simulink model "Question3cd"  (R2023b)
settings: Solver=VariableStepAuto  StartTime=0.0  StopTime=60.0  RelTol=1e-3
settings Model: Creator=akank  LastModifiedBy=akank

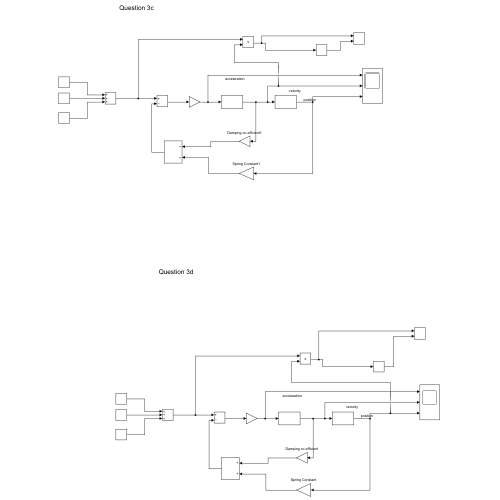
[thumbnail: Simulink's stored preview of the top-level diagram]
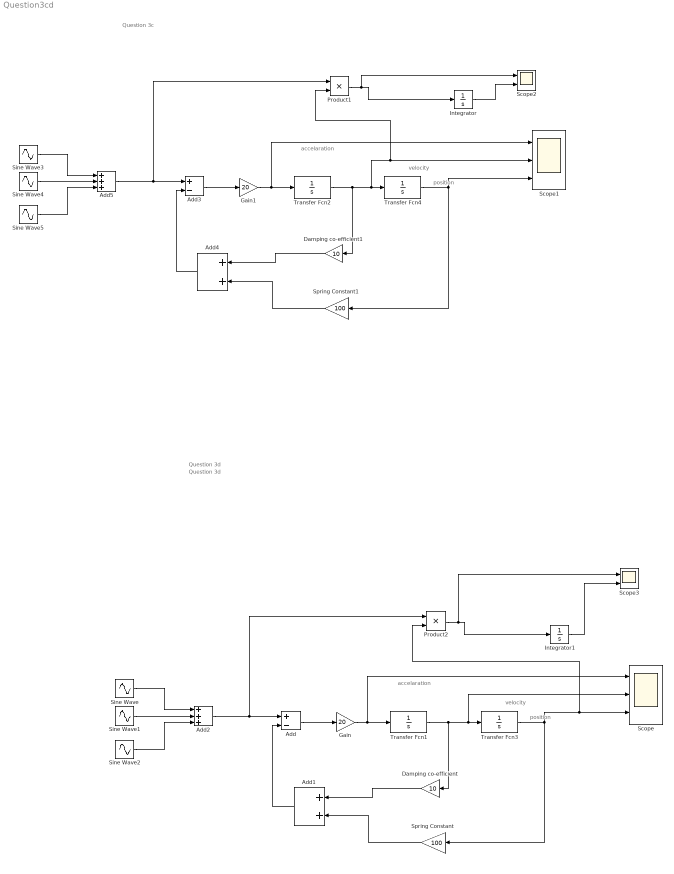
== system Question3cd ==
  note: Question 3c
  note: velocity
  note: accelaration
  note: position
  note: accelaration
  note: velocity
  note: position
  note: Question 3d
  note: Question 3d
  Add : Sum  Inputs=+-
  Add1 : Sum
  Add2 : Sum  Inputs=+++
  Add3 : Sum  Inputs=+-
  Add4 : Sum
  Add5 : Sum  Inputs=+++
  Damping co-efficient : Gain  Gain=10
  Damping co-efficient1 : Gain  Gain=10
  Gain : Gain  Gain=20
  Gain1 : Gain  Gain=20
  Integrator : Integrator  LimitOutput=on  LowerSaturationLimit=0
  Integrator1 : Integrator  LimitOutput=on  LowerSaturationLimit=0
  Product1 : Product
  Product2 : Product
  Scope : Scope  NumInputPorts=3
  Scope1 : Scope  NumInputPorts=3
  Scope2 : Scope  NumInputPorts=2
  Scope3 : Scope  NumInputPorts=2
  Sine Wave : Sin  Amplitude=20  SampleTime=0
  Sine Wave1 : Sin  Amplitude=10  Frequency=2.5  Phase=pi/2  SampleTime=0
  Sine Wave2 : Sin  Amplitude=20  Frequency=10  SampleTime=0
  Sine Wave3 : Sin  Amplitude=20  SampleTime=0
  Sine Wave4 : Sin  Amplitude=10  Frequency=2.5  Phase=pi/2  SampleTime=0
  Sine Wave5 : Sin  Amplitude=20  Frequency=10  SampleTime=0
  Spring Constant : Gain  Gain=100
  Spring Constant1 : Gain  Gain=100
  Transfer Fcn{1..4} (4 alike) : TransferFcn  Denominator=[1 0]
  wires:
  Spring Constant1/1 -> Add4/2
  Add4/1 -> Add3/2
  Add5/1 -> Product1/1, Add3/1
  Integrator/1 -> Scope2/2
  Sine Wave5/1 -> Add5/3
  Damping co-efficient1/1 -> Add4/1
  Sine Wave4/1 -> Add5/2
  Product1/1 -> Scope2/1, Integrator/1
  Gain1/1 -> Scope1/1, Transfer Fcn2/1
  Add3/1 -> Gain1/1
  Transfer Fcn4/1 -> Scope1/3, Spring Constant1/1
  Sine Wave3/1 -> Add5/1
  Transfer Fcn2/1 -> Product1/2, Scope1/2, Transfer Fcn4/1, Damping co-efficient1/1
  Sine Wave/1 -> Add2/1
  Add1/1 -> Add/2
  Damping co-efficient/1 -> Add1/1
  Transfer Fcn3/1 -> Product2/2, Scope/3, Spring Constant/1
  Spring Constant/1 -> Add1/2
  Add/1 -> Gain/1
  Product2/1 -> Scope3/1, Integrator1/1
  Sine Wave2/1 -> Add2/3
  Transfer Fcn1/1 -> Scope/2, Transfer Fcn3/1, Damping co-efficient/1
  Add2/1 -> Product2/1, Add/1
  Sine Wave1/1 -> Add2/2
  Integrator1/1 -> Scope3/2
  Gain/1 -> Scope/1, Transfer Fcn1/1
